simulink model "realize_filter"  (R2020b)
settings: Solver=VariableStepAuto  StartTime=0.0  StopTime=10  MaxStep=0.001  RelTol=1e-3
settings Model: Creator=vigne  LastModifiedBy=prabhudevmaddipudi

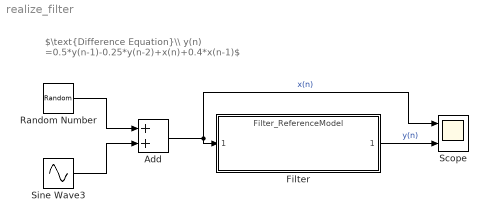
== system realize_filter ==
  note: $\text{Difference Equation}\\ y(n) =0.5*y(n-1)-0.25*y(n-2)+x(n)+0.4*x(n-1)$
  Add : Sum
  Filter : ModelReference  ModelNameDialog=Filter_ReferenceModel  SimulationMode=Normal  ModelReferenceVersion=1.10
  Random Number : RandomNumber  Variance=0.1  Seed=1  SampleTime=0.01
  Scope : Scope  NumInputPorts=2
  Sine Wave3 : Sin  Phase=2*pi*10000  SampleTime=0
  wires:
  Sine Wave3/1 -> Add/2
  Random Number/1 -> Add/1
  Add/1 -> Scope/1, Filter/1  "x(n)"
  Filter/1 -> Scope/2  "y(n)"
